simulink model "odev4_iremelmas_kara"  (R2023b)
settings: Solver=VariableStepAuto  StartTime=0.0  StopTime=2  MaxStep=1e-4  RelTol=1e-4
libraries: spsVoltageMeasurementLib x5, spsMeanLib x4, spsSeriesRLCBranchLib x3, spsCurrentMeasurementLib x3, spsDiodeLib x3, spsDCVoltageSourceLib x1, spsLinearTransformerLib x1, spsMosfetLib x1, spspowerguiLib x1
settings Model: Creator=ireme  LastModifiedBy=ireme

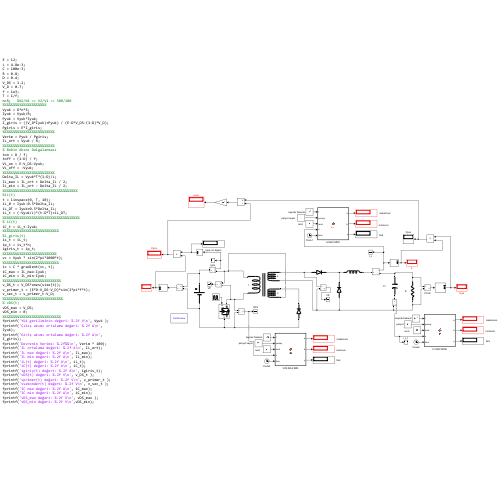
[thumbnail: Simulink's stored preview of the top-level diagram]
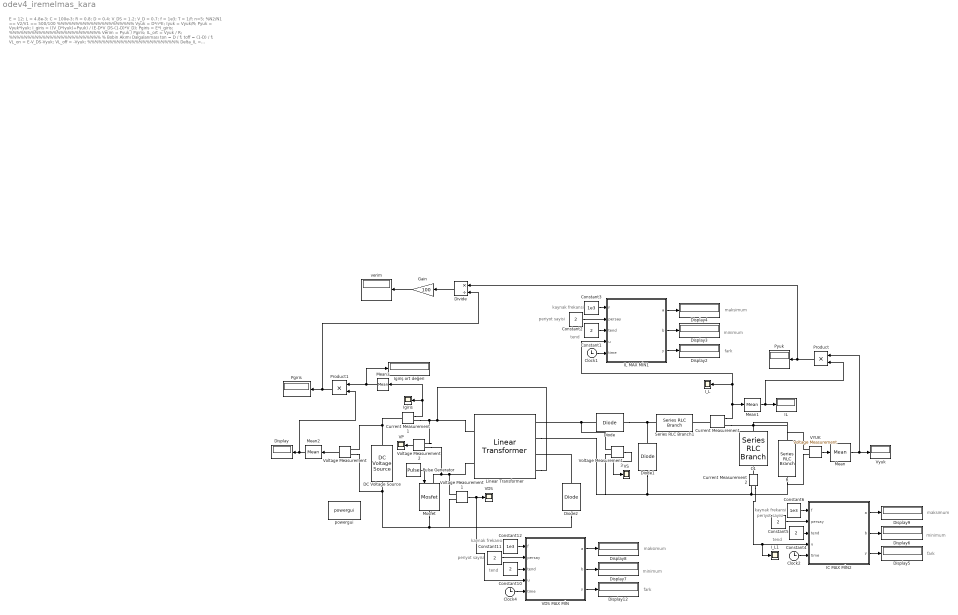
== system odev4_iremelmas_kara ==
  note: E = 12;
      | L = 4.8e-3;
      | C = 100e-3;
      | R = 0.8;
      | D = 0.4;
      | V_DS = 1.2;
      | V_D = 0.7;
      | f = 1e3;
      | T = 1/f;
      | n=5; %N2/N1 == V2/V1 == 500/100
      | %%%%%%%%%%%%%%%%%%%%%
      | Vyuk = D*n*E;
      | Iyuk = Vyuk/R;
      | Pyuk = Vyuk*Iyuk;
      | I_giris = ((V_D*Iyuk)+Pyuk) / (E-D*V_DS-(1-D)*V_D);
      | Pgiris = E*I_giris;
      | %%%%%%%%%%%%%%%%%%%%%%%%%
      | Verim = Pyuk / Pgiris;
      | IL_ort = Vyuk / R;
      | %%%%%%%%%%%%%%%%%%%%%%%%%
      | % Bobin Akımı Dalgalanması
      | ton = D / f;
      | toff = (1-D) / f;
      | VL_on = E-V_DS-Vyuk;
      | VL_off = -Vyuk;
      | %%%%%%%%%%%%%%%%%%%%%%%%%
      | Delta_IL = Vyuk*T*(1-D)/L;
      | IL_max = IL_ort + Delta_IL / 2;
      | IL_min = IL_ort - Delta_IL / 2;
      | %%%%%%%%%%%%%%%%%%%%%%%%%%%%%%%%%%%%
      | %iL(t)
      | t = linspace(0, T, 10);
      | iL_0 = Iyuk-0.5*Delta_IL;
      | iL_DT = Iyuk+0.5*Delta_IL;
      | iL_t = (-Vyuk/L)*(t-D*T)+iL_DT;
      | %%%%%%%%%%%%%%%%%%%%%%%%%%%%%%%%%%%%%
      | % iC(t)
      | iC_t = iL_t-Iyuk;
      | %%%%%%%%%%%%%%%%%%%%%%%%%%%
      | %i_giriş(t)
      | is_t = iL_t;
      | ip_t = is_t*n;
      | igiris_t = ip_t;
      | %%%%%%%%%%%%%%%%%%%%%%%%%%
      | vc = Vyuk * sin(2*pi*1000*t);
      | %%%%%%%%%%%%%%%%%%%%%%%%%%%
      | ic = C * gradient(vc, t);
      | iC_max = IL_max-Iyuk;
      | iC_min = IL_min-Iyuk;
      | %%%%%%%%%%%%%%%%%%%%%%%%%%%%
      | v_DS_t = V_DS*ones(size(t));
      | v_primer_t = (E*D-V_DS-V_D)*sin(2*pi*f*t);
      | v_sec_t = v_primer_t-V_D;
      | %%%%%%%%%%%%%%%%%%%%%%%%%%%%%
      | % vDS(t)
      | vDS_max = V_DS;
      | vDS_min = 0;
      | %%%%%%%%%%%%%%%%%%%%%%%%%%%%
      | fprintf( 'Yük geriliminin değeri: %.2f V\n' , Vyuk );
      | fprintf( 'Çıkış akımı ortalama değeri: %.2f A\n' , Iyuk);
      | fprintf( 'Giriş akımı ortalama değeri: %.2f A\n' , I_giris);
      | fprintf( 'Devrenin Verimi: %.2f%%\n' , Verim * 100);
      | fprintf( 'IL ortalama değeri: %.2f A\n' , IL_ort);
      | fprintf( 'IL max değeri: %.2f A\n' , IL_max);
      | fprintf( 'IL min değeri: %.2f A\n' , IL_min);
      | fprintf( 'iL(t) değeri: %.2f A\n' , iL_t);
      | fprintf( 'iC(t) değeri: %.2f A\n' , iC_t);
      | fprintf( 'igiriş(t) değeri: %.2f A\n' , igiris_t);
      | fprintf( 'vDS(t) değeri: %.2f V\n' , v_DS_t );
      | fprintf( 'vprimer(t) değeri: %.2f V\n' , v_primer_t );
      | fprintf( 'vsekonder(t) değeri: %.2f V\n' , v_sec_t );
      | fprintf( 'IC max değeri: %.2f A\n' , iC_max);
      | fprintf( 'IC min değeri: %.2f A\n' , iC_min);
      | fprintf( 'vDS_max değeri: %.2f V\n' , vDS_max );
      | fprintf( 'vDS_min değeri: %.2f V\n' ,vDS_min);
  note: maksimum
  note: kaynak frekansi
  note: minimum
  note: tend
  note: periyot sayisi
  note: fark
  note: periyot sayisi
  note: kaynak frekansi
  note: maksimum
  note: fark
  note: minimum
  note: tend
  note: periyot sayisi
  note: kaynak frekansi
  note: maksimum
  note: fark
  note: minimum
  note: tend
  C1 : spsSeriesRLCBranchLib/Series RLC Branch  LConnTagsString=__new0  RConnTagsString=__new0  BranchType=C  Resistance=1  Inductance=180e-6  SetiL0=off  InitialCurrent=0  Capacitance=100e-3  Setx0=off  InitialVoltage=0  Measurements=None
  Clock1 : Clock
      settings: Decimation=100
  Clock2 : Clock
      settings: Decimation=100
  Clock4 : Clock
      settings: Decimation=100
  Constant{1..2,4..5,10..11} (6 alike) : Constant  Value=2  SampleTime=0
  Constant12 : Constant  Value=1e3  SampleTime=0
  Constant3 : Constant  Value=1e3  SampleTime=0
  Constant6 : Constant  Value=1e3  SampleTime=0
  Current Measurement : spsCurrentMeasurementLib/Current Measurement  PhasorSimulation=off  OutputType=Complex  PSBequivalent=0
  Current Measurement1 : spsCurrentMeasurementLib/Current Measurement  PhasorSimulation=off  OutputType=Complex  PSBequivalent=0
  Current Measurement2 : spsCurrentMeasurementLib/Current Measurement  PhasorSimulation=off  OutputType=Complex  PSBequivalent=0
  DC Voltage Source : spsDCVoltageSourceLib/DC Voltage Source  Amplitude=12  Measurements=None
  Diode : spsDiodeLib/Diode  Ron=1e-8  Lon=0  Vf=0.7  IC=0  UseSnubber=0  Rs=inf  Cs=0  Measurements=off
  Diode1 : spsDiodeLib/Diode  Ron=1e-8  Lon=0  Vf=0.7  IC=0  UseSnubber=0  Rs=inf  Cs=0  Measurements=off
  Diode2 : spsDiodeLib/Diode  Ron=1e-8  Lon=0  Vf=0.7  IC=0  UseSnubber=0  Rs=inf  Cs=0  Measurements=off
  Display{,2..9,12} (10 alike) : Display
  Divide : Product  Inputs=*/
  Gain : Gain  Gain=100
  IC MAX MİN2 : MATLAB Function  TreatAsAtomicUnit=on
  IL : Display
  IL MAX MİN1 : MATLAB Function  TreatAsAtomicUnit=on
  I_L : Scope
  I_L1 : Scope
  Igiris : Scope
  Igiriş ort değeri : Display
  Linear Transformer : spsLinearTransformerLib/Linear Transformer  UNITS=SI  NominalPower=[1000 1e3]  winding1=[100 0 0]  winding2=[500 0 0]  ThreeWindings=on  winding3=[100 0 0]  RmLm=[inf 1e-3]  Measurements=Magnetization current  DataType=on
  Mean{,1..3} (4 alike) : spsMeanLib/Mean  Freq=1e3  Vinit=0  Ts=0
  Mosfet : spsMosfetLib/Mosfet  Ron=1e-8  Lon=0  Rd=1e-8  Vfd=1.2  IC=0  Rs=1e6  Cs=inf  Measurements=off
  Pgiris : Display
  Product : Product
  Product1 : Product
  Pulse Generator : DiscretePulseGenerator  PulseType=Time based  Period=1e-3  PulseWidth=40
  Pyuk : Display
  R : spsSeriesRLCBranchLib/Series RLC Branch  LConnTagsString=__new0  RConnTagsString=__new0  BranchType=R  Resistance=0.8  Inductance=180e-6  SetiL0=off  InitialCurrent=0  Capacitance=1e-6  Setx0=off  InitialVoltage=0  Measurements=None
  Series RLC Branch1 : spsSeriesRLCBranchLib/Series RLC Branch  LConnTagsString=__new0  RConnTagsString=__new0  BranchType=L  Resistance=1  Inductance=4.8e-3  SetiL0=off  InitialCurrent=0  Capacitance=1e-6  Setx0=off  InitialVoltage=0  Measurements=None
  VDS : Scope
  VDS MAX MİN : MATLAB Function  TreatAsAtomicUnit=on
  VP : Scope
  VS : Scope
  VYUK : spsVoltageMeasurementLib/Voltage Measurement  PhasorSimulation=off  OutputType=Complex  PSBequivalent=0
  Voltage Measurement{,1..3} (4 alike) : spsVoltageMeasurementLib/Voltage Measurement  PhasorSimulation=off  OutputType=Complex  PSBequivalent=0
  Vyuk : Display
  powergui : spspowerguiLib/powergui  Priority=1  SimulationMode=Continuous  SampleTime=50e-8  frequency=60  Iterations=50  frequencyindice=0  Pbase=100e6  ErrMax=1e-4  UnitsV=kV  UnitsW=MW  buscounter=0  FunctionMessages=off  echomessages=off  EnableUseOfTLC=off  CurrentSourceSwitches=off  DisableSnubberDevices=on  DisableRonSwitches=on  DisableVfSwitches=off  DisplayEquations=off  AutomaticDiscreteSolvers=off  SolverType=Tustin/Backward Euler (TBE)  Interpol=off  ExternalGateDelay=off  methode=off  Ts=100  x0status=zero  SPID=off  SwTol=0  HookPort=off  NonlinearTolerance=0  nMaxIteration=15  ContinueOnMaxIteration=off  RestoreLinks=warning  ResistiveCurrentMeasurement=off  Frange=[0:2:500]  Ylog=off  Xlog=on  ShowGrid=off  save=off  variable=ZData  structure=0  ZoomFFT=off  StartTime=0.0  cycles=1  DisplayStyle=1  fundamental=60  FreqAxis=off  MaxFrequency=1000  frequencyindicesteady=1  RmsSteady=1  display=off
  verim : Display
  wires:
  Pulse Generator/1 -> Mosfet/1
  Mean/1 -> Product/1, Vyuk/1
  VYUK/1 -> Mean/1
  Current Measurement/1 -> IL MAX MİN1/4(u), I_L/1, Mean1/1
  Mean1/1 -> Product/2, IL/1
  Product/1 -> Divide/1, Pyuk/1
  Voltage Measurement/1 -> Mean2/1
  Mean2/1 -> Product1/2, Display/1
  Product1/1 -> Divide/2, Pgiris/1
  Divide/1 -> Gain/1
  Gain/1 -> verim/1
  Current Measurement1/1 -> Igiris/1, Mean3/1
  Current Measurement2/1 -> I_L1/1, IC MAX MİN2/4(u)
  Voltage Measurement1/1 -> VDS/1, VDS MAX MİN/4(u)
  Voltage Measurement2/1 -> VP/1
  Voltage Measurement3/1 -> VS/1
  Constant11/1 -> VDS MAX MİN/2(persay)
  Clock4/1 -> VDS MAX MİN/5(time)
  VDS MAX MİN/2(b) -> Display7/1
  VDS MAX MİN/3(y) -> Display12/1
  VDS MAX MİN/1(a) -> Display8/1
  Constant12/1 -> VDS MAX MİN/1(f)
  Constant10/1 -> VDS MAX MİN/3(tend)
  Clock1/1 -> IL MAX MİN1/5(time)
  Constant3/1 -> IL MAX MİN1/1(f)
  Constant1/1 -> IL MAX MİN1/3(tend)
  IL MAX MİN1/3(y) -> Display2/1
  Constant2/1 -> IL MAX MİN1/2(persay)
  IL MAX MİN1/2(b) -> Display3/1
  IL MAX MİN1/1(a) -> Display4/1
  Clock2/1 -> IC MAX MİN2/5(time)
  Constant6/1 -> IC MAX MİN2/1(f)
  Constant4/1 -> IC MAX MİN2/3(tend)
  IC MAX MİN2/3(y) -> Display5/1
  Constant5/1 -> IC MAX MİN2/2(persay)
  IC MAX MİN2/2(b) -> Display6/1
  IC MAX MİN2/1(a) -> Display9/1
  Mean3/1 -> Igiriş ort değeri/1, Product1/1
  connections:
  Series RLC Branch1/LConn1 -- Diode1/RConn1 -- Diode/RConn1
  VYUK/LConn1 -- R/LConn1 -- Current Measurement/RConn1 -- C1/LConn1
  DC Voltage Source/RConn1 -- Current Measurement1/LConn1 -- Voltage Measurement/LConn1
  Mosfet/LConn1 -- Voltage Measurement2/LConn2 -- Voltage Measurement1/LConn1 -- Linear Transformer/LConn2
  Mosfet/RConn1 -- Voltage Measurement1/LConn2 -- Diode2/LConn1 -- Voltage Measurement/LConn2 -- DC Voltage Source/LConn1
  VYUK/LConn2 -- R/RConn1 -- Current Measurement2/RConn1 -- Voltage Measurement3/LConn2 -- Linear Transformer/RConn2 -- Diode1/LConn1
  Current Measurement/LConn1 -- Series RLC Branch1/RConn1
  Current Measurement1/RConn1 -- Voltage Measurement2/LConn1 -- Linear Transformer/LConn1 -- Linear Transformer/RConn4
  Diode/LConn1 -- Voltage Measurement3/LConn1 -- Linear Transformer/RConn1
  Diode2/RConn1 -- Linear Transformer/RConn3
  Current Measurement2/LConn1 -- C1/RConn1

== matlab function odev4_iremelmas_kara/IL MAX MİN1 ==
  settings: updateMethod=DISCRETE
  data: a output; b output; f input; persay input; tend input; u input; y output; time input
function [a,b,y] = fcn(f,persay,tend,u,time)
% persistent değişken; değişken değerini kalıcı olarak tutar ve direk atama
% yapılmadıkça değişmez. Normal değişkenler fonksiyonun her yenilenme 
% durumunda sıfırlanırken, persistent değişkeni, kalıcı olması sebebiyle,
% bir önceki değeri tutabilme yeteneğine sahiptir. 
% Bu da bize bir önceki değer ile güncel değerinizi karşılaştırma olanağı
% sunar.
a=1/0;b=0;
persistent enbuyuk;
persistent enkucuk;
persistent fark;
% Eğer persistent değişkenini en başta persistent enbuyuk = 0; olarak 
% tanımlarsak, sürekli 0 olarak kalacaktır. Aynı zamanda eğer bir ilk değer 
% vermezseniz "null" değerini taşıyacağından, if yapılarında hata
% verecektir. Bu hatadan kaçınmak için, isempty komutu ile persistent
% değişkenlerinin "null" olup olmadığını kontrol edilir ve ilk değer ataması
% yapılır. Bu değişkenler sadece  fonksiyon ilk kez çalıştığında
% null olacağı için(daha sonra sürekli gelen değeri tuttuğu yukarıda söylenmişti)
% başlangıçta, bir kereye mahsus olarak,  aşağıdaki if yapısı doğrulanacak 
% ve değişkenlere ilk değerler atanacaktır.
%
if (isempty(enkucuk) || isempty(enbuyuk))  
enkucuk = 1/0;   
enbuyuk = 0;
end
if (time>tend-(persay+1)*1/f) && (time<=tend) % Periyot ~= 0.01 // Son iki periyodu hesaplar.
    if u >= enbuyuk
        enbuyuk = u;
     end
    if u < enkucuk   
        enkucuk = u;
    end
end
fark = enbuyuk - enkucuk;
a=enbuyuk;
b=enkucuk;
y=fark;
end

== matlab function odev4_iremelmas_kara/IC MAX MİN2 ==
  settings: updateMethod=DISCRETE
  data: a output; b output; f input; persay input; tend input; u input; y output; time input
function [a,b,y] = fcn(f,persay,tend,u,time)
% persistent değişken; değişken değerini kalıcı olarak tutar ve direk atama
% yapılmadıkça değişmez. Normal değişkenler fonksiyonun her yenilenme 
% durumunda sıfırlanırken, persistent değişkeni, kalıcı olması sebebiyle,
% bir önceki değeri tutabilme yeteneğine sahiptir. 
% Bu da bize bir önceki değer ile güncel değerinizi karşılaştırma olanağı
% sunar.
a=1/0;b=0;
persistent enbuyuk;
persistent enkucuk;
persistent fark;
% Eğer persistent değişkenini en başta persistent enbuyuk = 0; olarak 
% tanımlarsak, sürekli 0 olarak kalacaktır. Aynı zamanda eğer bir ilk değer 
% vermezseniz "null" değerini taşıyacağından, if yapılarında hata
% verecektir. Bu hatadan kaçınmak için, isempty komutu ile persistent
% değişkenlerinin "null" olup olmadığını kontrol edilir ve ilk değer ataması
% yapılır. Bu değişkenler sadece  fonksiyon ilk kez çalıştığında
% null olacağı için(daha sonra sürekli gelen değeri tuttuğu yukarıda söylenmişti)
% başlangıçta, bir kereye mahsus olarak,  aşağıdaki if yapısı doğrulanacak 
% ve değişkenlere ilk değerler atanacaktır.
%
if (isempty(enkucuk) || isempty(enbuyuk))  
enkucuk = 1/0;   
enbuyuk = 0;
end
if (time>tend-(persay+1)*1/f) && (time<=tend) % Periyot ~= 0.01 // Son iki periyodu hesaplar.
    if u >= enbuyuk
        enbuyuk = u;
     end
    if u < enkucuk   
        enkucuk = u;
    end
end
fark = enbuyuk - enkucuk;
a=enbuyuk;
b=enkucuk;
y=fark;
end

== matlab function odev4_iremelmas_kara/VDS MAX MİN ==
  settings: updateMethod=DISCRETE
  data: a output; b output; f input; persay input; tend input; u input; y output; time input
function [a,b,y] = fcn(f,persay,tend,u,time)
% persistent değişken; değişken değerini kalıcı olarak tutar ve direk atama
% yapılmadıkça değişmez. Normal değişkenler fonksiyonun her yenilenme 
% durumunda sıfırlanırken, persistent değişkeni, kalıcı olması sebebiyle,
% bir önceki değeri tutabilme yeteneğine sahiptir. 
% Bu da bize bir önceki değer ile güncel değerinizi karşılaştırma olanağı
% sunar.
a=1/0;b=0;
persistent enbuyuk;
persistent enkucuk;
persistent fark;
% Eğer persistent değişkenini en başta persistent enbuyuk = 0; olarak 
% tanımlarsak, sürekli 0 olarak kalacaktır. Aynı zamanda eğer bir ilk değer 
% vermezseniz "null" değerini taşıyacağından, if yapılarında hata
% verecektir. Bu hatadan kaçınmak için, isempty komutu ile persistent
% değişkenlerinin "null" olup olmadığını kontrol edilir ve ilk değer ataması
% yapılır. Bu değişkenler sadece  fonksiyon ilk kez çalıştığında
% null olacağı için(daha sonra sürekli gelen değeri tuttuğu yukarıda söylenmişti)
% başlangıçta, bir kereye mahsus olarak,  aşağıdaki if yapısı doğrulanacak 
% ve değişkenlere ilk değerler atanacaktır.
%
if (isempty(enkucuk) || isempty(enbuyuk))  
enkucuk = 1/0;   
enbuyuk = 0;
end
if (time>tend-(persay+1)*1/f) && (time<=tend) % Periyot ~= 0.01 // Son iki periyodu hesaplar.
    if u >= enbuyuk
        enbuyuk = u;
     end
    if u < enkucuk   
        enkucuk = u;
    end
end
fark = enbuyuk - enkucuk;
a=enbuyuk;
b=enkucuk;
y=fark;
end
